simulink model "LQR_discrete"  (R2014b)
settings: Solver=ode45  StartTime=0.0  StopTime=T_sim  RelTol=1e-3
values from neighbouring files (symbols this model uses):
  set_point = [0; 0; 0; 0]    [cessna.m]
  sys_discrete = c2d(sys, Ts)    [cessna.m]
  Ts = 0.1    [cessna.m]
  u_max_simulink = inf    [cessna.m]
  u_min_simulink = -inf    [cessna.m]
  x0 = [0; 0; 0; 10]    [cessna.m]
undefined symbols (not defined in the file or in its folder): Kdlqr
settings Model: Creator=lele  LastModifiedBy=lele

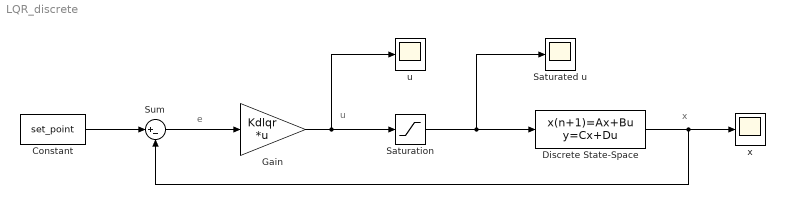
== system LQR_discrete ==
  note: x
  note: u
  note: e
  Constant : Constant  Value=set_point
  Discrete State-Space : DiscreteStateSpace  A=sys_discrete.a  B=sys_discrete.b  C=eye(4)  D=zeros(4, 1)  X0=x0  SampleTime=Ts
  Gain : Gain  Gain=Kdlqr  Multiplication=Matrix(K*u)
  Saturated u : Scope
      settings: SaveName=ScopeData2
  Saturation : Saturate  UpperLimit=u_max_simulink  LowerLimit=u_min_simulink
  Sum : Sum  Inputs=|+-
  u : Scope
  x : Scope
      settings: ShowLegends=on
  wires:
  Constant/1 -> Sum/1
  Sum/1 -> Gain/1
  Discrete State-Space/1 -> Sum/2, x/1
  Gain/1 -> u/1, Saturation/1
  Saturation/1 -> Discrete State-Space/1, Saturated u/1
